simulink model "Almost_there"  (R2022a)
settings: Solver=FixedStepAuto  StartTime=0.0  StopTime=10.0  RelTol=1e-3  EnableMultiTasking=on
undefined symbols (not defined in the file): InputPWM, ticksPerRot, wheelR, WheelSpeed
libraries: arduinolib x19, spsEdgeDetectorLib x2, mobileRoboticsTrainingLib x1
settings Model: ExtModeTrigDuration=2  Creator=heath  LastModifiedBy=noahhavik
settings OptimizationCC: EnhancedBackFolding=on  PassReuseOutputArgsAs=Individual arguments  ZeroExternalMemoryAtStartup=off  ZeroInternalMemoryAtStartup=off  MaxStackSize=64  OptimizeBlockOrder=speed  DifferentSizesBufferReuse=on  OptimizationCustomize=off  EfficientTunableParamExpr=on
settings DebuggingCC: MultiTaskDSMMsg=none  ParameterTunabilityLossMsg=error
settings HardwareCC: ProdBitPerPointer=32  ProdBitPerSizeT=32  ProdBitPerPtrDiffT=32  ProdLargestAtomicInteger=Long  ProdLargestAtomicFloat=Double  ProdWordSize=32  ProdHWDeviceType=ARM Compatible->ARM Cortex  UseEmbeddedCoderFeatures=off  UseSimulinkCoderFeatures=off
settings SFSimCC: MATLABDynamicMemAlloc=off
settings RTWCC: SystemTargetFile=ert.tlc  HardwareBoard=Arduino Nano 33 IoT  TemplateMakefile=ert_default_tmf  Toolchain=Arduino ARM  BuildConfiguration=Faster Runs
settings CodeAppCC: ForceParamTrailComments=on  IgnoreCustomStorageClasses=off  OperatorAnnotations=on  SimulinkDataObjDesc=on  SFDataObjDesc=on  InsertBlockDesc=on
settings ERTTargetCC: SupportContinuousTime=on  SupportNonInlinedSFcns=on  SupportVariableSizeSignals=on  ExtModeTransport=3  ExtModeStaticAlloc=on  ExtModeStaticAllocSize=8192  ExtModeMexFile=ext_xcp  ExtModeIntrfLevel=Level2 - Open

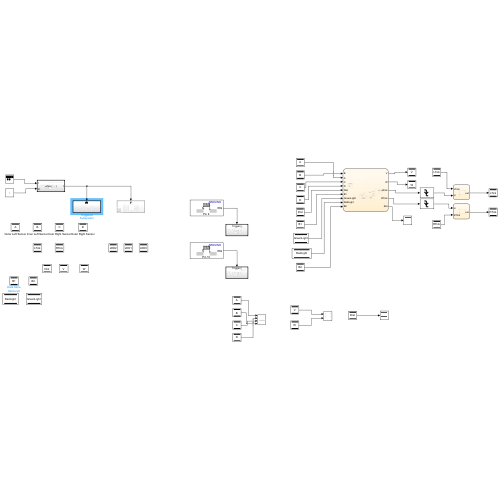
[thumbnail: Simulink's stored preview of the top-level diagram]
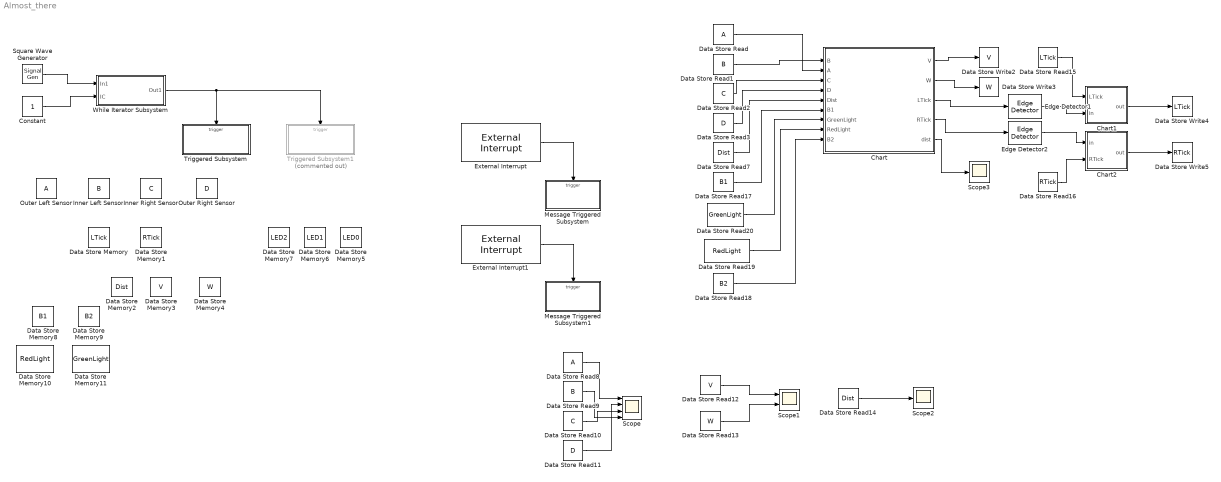
== system Almost_there ==
  Chart : Stateflow chart  TreatAsAtomicUnit=on
  Chart1 : Stateflow chart  TreatAsAtomicUnit=on
  Chart2 : Stateflow chart  TreatAsAtomicUnit=on
  Constant : Constant
  Data Store Memory : DataStoreMemory  DataStoreName=LTick  ShowAdditionalParam=off
  Data Store Memory1 : DataStoreMemory  DataStoreName=RTick  WriteAfterWriteMsg=warning  ShowAdditionalParam=off
  Data Store Memory10 : DataStoreMemory  DataStoreName=RedLight  WriteAfterWriteMsg=warning  ShowAdditionalParam=off
  Data Store Memory11 : DataStoreMemory  DataStoreName=GreenLight  WriteAfterWriteMsg=warning  ShowAdditionalParam=off
  Data Store Memory2 : DataStoreMemory  DataStoreName=Dist  WriteAfterWriteMsg=warning  ShowAdditionalParam=off
  Data Store Memory3 : DataStoreMemory  DataStoreName=V  WriteAfterWriteMsg=warning  ShowAdditionalParam=off
  Data Store Memory4 : DataStoreMemory  DataStoreName=W  WriteAfterWriteMsg=warning  ShowAdditionalParam=off
  Data Store Memory5 : DataStoreMemory  DataStoreName=LED0  WriteAfterWriteMsg=warning  ShowAdditionalParam=off
  Data Store Memory6 : DataStoreMemory  DataStoreName=LED1  WriteAfterWriteMsg=warning  ShowAdditionalParam=off
  Data Store Memory7 : DataStoreMemory  DataStoreName=LED2  WriteAfterWriteMsg=warning  ShowAdditionalParam=off
  Data Store Memory8 : DataStoreMemory  DataStoreName=B1  WriteAfterWriteMsg=warning  ShowAdditionalParam=off
  Data Store Memory9 : DataStoreMemory  DataStoreName=B2  WriteAfterWriteMsg=warning  ShowAdditionalParam=off
  Data Store Read : DataStoreRead  IndexOptions=Index vector (dialog)  Indices=1  OutputSizes=1
  Data Store Read1 : DataStoreRead  DataStoreName=B  IndexOptions=Index vector (dialog)  Indices=1  OutputSizes=1
  Data Store Read10 : DataStoreRead  DataStoreName=C  IndexOptions=Index vector (dialog)  Indices=1  OutputSizes=1
  Data Store Read11 : DataStoreRead  DataStoreName=D  IndexOptions=Index vector (dialog)  Indices=1  OutputSizes=1
  Data Store Read12 : DataStoreRead  DataStoreName=V  IndexOptions=Index vector (dialog)  Indices=1  OutputSizes=1
  Data Store Read13 : DataStoreRead  DataStoreName=W  IndexOptions=Index vector (dialog)  Indices=1  OutputSizes=1
  Data Store Read14 : DataStoreRead  DataStoreName=Dist  IndexOptions=Index vector (dialog)  Indices=1  OutputSizes=1
  Data Store Read15 : DataStoreRead  DataStoreName=LTick  IndexOptions=Index vector (dialog)  Indices=1  OutputSizes=1
  Data Store Read16 : DataStoreRead  DataStoreName=RTick  IndexOptions=Index vector (dialog)  Indices=1  OutputSizes=1
  Data Store Read17 : DataStoreRead  DataStoreName=B1  IndexOptions=Index vector (dialog)  Indices=1  OutputSizes=1
  Data Store Read18 : DataStoreRead  DataStoreName=B2  IndexOptions=Index vector (dialog)  Indices=1  OutputSizes=1
  Data Store Read19 : DataStoreRead  DataStoreName=RedLight  IndexOptions=Index vector (dialog)  Indices=1  OutputSizes=1
  Data Store Read2 : DataStoreRead  DataStoreName=C  IndexOptions=Index vector (dialog)  Indices=1  OutputSizes=1
  Data Store Read20 : DataStoreRead  DataStoreName=GreenLight  IndexOptions=Index vector (dialog)  Indices=1  OutputSizes=1
  Data Store Read3 : DataStoreRead  DataStoreName=D  IndexOptions=Index vector (dialog)  Indices=1  OutputSizes=1
  Data Store Read7 : DataStoreRead  DataStoreName=Dist  IndexOptions=Index vector (dialog)  Indices=1  OutputSizes=1
  Data Store Read8 : DataStoreRead  IndexOptions=Index vector (dialog)  Indices=1  OutputSizes=1
  Data Store Read9 : DataStoreRead  DataStoreName=B  IndexOptions=Index vector (dialog)  Indices=1  OutputSizes=1
  Data Store Write2 : DataStoreWrite  DataStoreName=V  IndexOptions=Index vector (dialog)  Indices=1  OutputSizes=1
  Data Store Write3 : DataStoreWrite  DataStoreName=W  IndexOptions=Index vector (dialog)  Indices=1  OutputSizes=1
  Data Store Write4 : DataStoreWrite  DataStoreName=LTick  IndexOptions=Index vector (dialog)  Indices=1  OutputSizes=1
  Data Store Write5 : DataStoreWrite  DataStoreName=RTick  IndexOptions=Index vector (dialog)  Indices=1  OutputSizes=1
  Edge Detector1 : spsEdgeDetectorLib/Edge Detector  model=Falling  ic=0  Ts=0
      settings: SourceProductBaseCode=PS
  Edge Detector2 : spsEdgeDetectorLib/Edge Detector  model=Falling  ic=0  Ts=0
      settings: SourceProductBaseCode=PS
  External Interrupt : arduinolib/External Interrupt  Pin=9  PullUp=off  Mode=RISING  InterruptSimulationInput=off
      settings: SourceProductBaseCode=ARDUINO
  External Interrupt1 : arduinolib/External Interrupt  Pin=10  PullUp=off  Mode=RISING  InterruptSimulationInput=off
      settings: SourceProductBaseCode=ARDUINO
  Inner Left Sensor : DataStoreMemory  DataStoreName=B  WriteAfterWriteMsg=warning  ShowAdditionalParam=off
  Inner Right Sensor : DataStoreMemory  DataStoreName=C  WriteAfterWriteMsg=warning  ShowAdditionalParam=off
  Message Triggered Subsystem : Subsystem  TreatAsAtomicUnit=on
  Message Triggered Subsystem1 : Subsystem  TreatAsAtomicUnit=on
  Outer Left Sensor : DataStoreMemory  WriteAfterWriteMsg=warning  ShowAdditionalParam=off
  Outer Right Sensor : DataStoreMemory  DataStoreName=D  WriteAfterWriteMsg=warning  ShowAdditionalParam=off
  Scope : Scope  NumInputPorts=4
  Scope1 : Scope  NumInputPorts=2
  Scope2 : Scope
  Scope3 : Scope
  Square Wave Generator : SignalGenerator  WaveForm=square  Frequency=100
  Triggered Subsystem : Subsystem  TreatAsAtomicUnit=on
  Triggered Subsystem1 : Subsystem  Commented=on  TreatAsAtomicUnit=on
  While Iterator Subsystem : Subsystem  TreatAsAtomicUnit=on
  wires:
  Square Wave Generator/1 -> While Iterator Subsystem/1(In1)
  Constant/1 -> While Iterator Subsystem/2(IC)
  External Interrupt/1 -> Message Triggered Subsystem/Trigger
  External Interrupt1/1 -> Message Triggered Subsystem1/Trigger
  While Iterator Subsystem/1(Out1) -> Triggered Subsystem/Trigger, Triggered Subsystem1/Trigger
  Chart/1(V) -> Data Store Write2/1
  Data Store Read7/1 -> Chart/5(Dist)
  Data Store Read3/1 -> Chart/4(D)
  Data Store Read2/1 -> Chart/3(C)
  Data Store Read1/1 -> Chart/1(B)
  Chart/2(W) -> Data Store Write3/1
  Data Store Read/1 -> Chart/2(A)
  Data Store Read8/1 -> Scope/1
  Data Store Read9/1 -> Scope/4
  Data Store Read10/1 -> Scope/3
  Data Store Read11/1 -> Scope/2
  Data Store Read12/1 -> Scope1/1
  Data Store Read13/1 -> Scope1/2
  Data Store Read14/1 -> Scope2/1
  Chart/3(LTick) -> Edge Detector1/1
  Edge Detector1/1 -> Chart1/2(in)
  Chart1/1(out) -> Data Store Write4/1
  Data Store Read15/1 -> Chart1/1(LTick)
  Chart2/1(out) -> Data Store Write5/1
  Edge Detector2/1 -> Chart2/1(in)
  Chart/4(RTick) -> Edge Detector2/1
  Data Store Read16/1 -> Chart2/2(RTick)
  Chart/5(dist) -> Scope3/1
  Data Store Read17/1 -> Chart/6(B1)
  Data Store Read20/1 -> Chart/7(GreenLight)
  Data Store Read19/1 -> Chart/8(RedLight)
  Data Store Read18/1 -> Chart/9(B2)

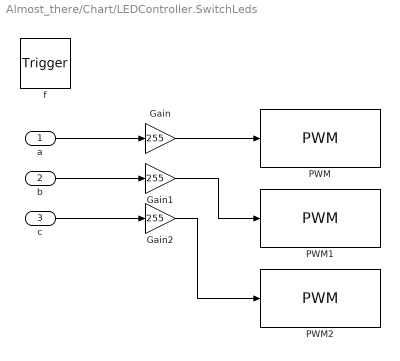
== system Almost_there/Chart/LEDController.SwitchLeds ==
  a : Inport  OutDataTypeStr=double  PortDimensions=1
  b : Inport  Port=2  OutDataTypeStr=double  PortDimensions=1
  c : Inport  Port=3  OutDataTypeStr=double  PortDimensions=1
  f : TriggerPort  TriggerType=function-call  VariantControl=(inherit)
      settings: CopyFcn=Stateflow.SLINSF.SimulinkMan.removeBlockPreDeleteFcn  PreDeleteFcn=Stateflow.SLINSF.SimulinkMan.unsafePredeleteFcn
  Gain : Gain  Gain=255
  Gain1 : Gain  Gain=255
  Gain2 : Gain  Gain=255
  PWM : arduinolib/PWM  pinNumber=16  frequencyType=Default  desiredFrequency=490.2  achievableFrequency=490.2
  PWM1 : arduinolib/PWM  pinNumber=17  frequencyType=Default  desiredFrequency=490.2  achievableFrequency=490.2
  PWM2 : arduinolib/PWM  pinNumber=19  frequencyType=Default  desiredFrequency=490.2  achievableFrequency=490.2
  wires:
  Gain/1 -> PWM/1
  Gain1/1 -> PWM1/1
  Gain2/1 -> PWM2/1
  a/1 -> Gain/1
  b/1 -> Gain1/1
  c/1 -> Gain2/1

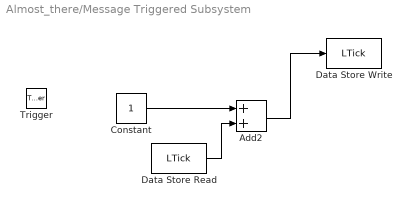
== system Almost_there/Message Triggered Subsystem ==
  Trigger : TriggerPort  TriggerType=function-call  VariantControl=(inherit)  PortDimensions=1
  Add2 : Sum
  Constant : Constant
  Data Store Read : DataStoreRead  DataStoreName=LTick  IndexOptions=Index vector (dialog)  Indices=1  OutputSizes=1
  Data Store Write : DataStoreWrite  DataStoreName=LTick  IndexOptions=Index vector (dialog)  Indices=1  OutputSizes=1
  wires:
  Add2/1 -> Data Store Write/1
  Constant/1 -> Add2/1
  Data Store Read/1 -> Add2/2

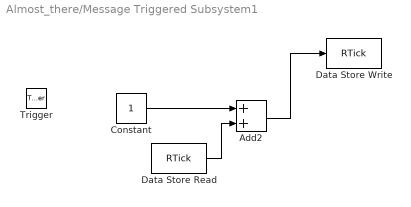
== system Almost_there/Message Triggered Subsystem1 ==
  Trigger : TriggerPort  TriggerType=function-call  VariantControl=(inherit)  PortDimensions=1
  Add2 : Sum
  Constant : Constant
  Data Store Read : DataStoreRead  DataStoreName=RTick  IndexOptions=Index vector (dialog)  Indices=1  OutputSizes=1
  Data Store Write : DataStoreWrite  DataStoreName=RTick  IndexOptions=Index vector (dialog)  Indices=1  OutputSizes=1
  wires:
  Add2/1 -> Data Store Write/1
  Constant/1 -> Add2/1
  Data Store Read/1 -> Add2/2

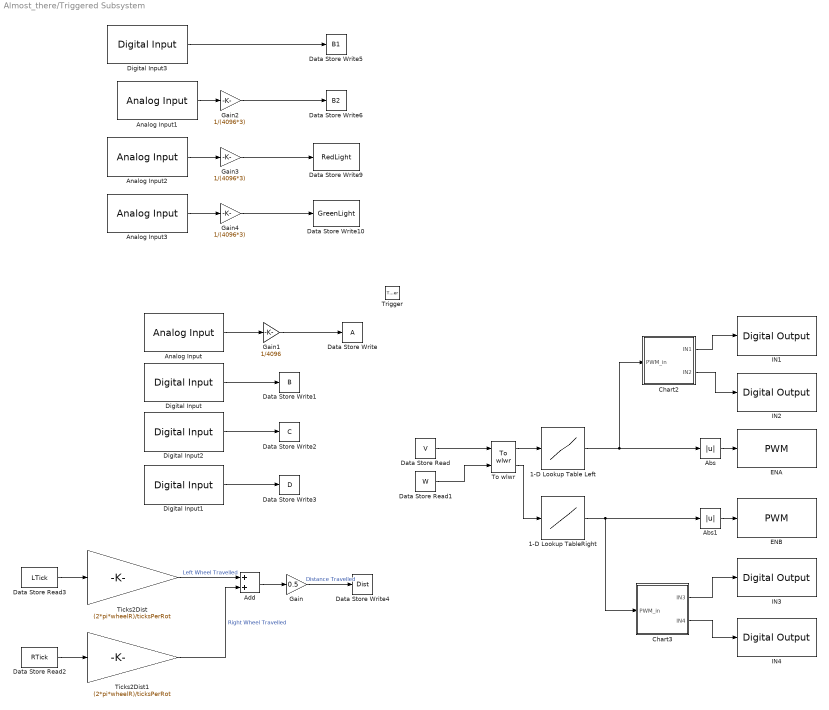
== system Almost_there/Triggered Subsystem ==
  Trigger : TriggerPort  TriggerType=either  VariantControl=(inherit)
  1-D Lookup Table Left : Lookup_n-D  NumberOfTableDimensions=1  BreakpointsForDimension1=WheelSpeed  Table=InputPWM  InternalRulePriority=Speed  RndMeth=Simplest
  1-D Lookup TableRight : Lookup_n-D  NumberOfTableDimensions=1  BreakpointsForDimension1=WheelSpeed  Table=InputPWM  InternalRulePriority=Speed  RndMeth=Simplest
  Abs : Abs  SaturateOnIntegerOverflow=off
  Abs1 : Abs  SaturateOnIntegerOverflow=off
  Add : Sum
  Analog Input : arduinolib/Analog Input  pinNumber=0  ReadResultsOnly=off  ConversionTriggerSource=Software  ExternalTriggerType=uint32( 0 )  OutputDataType=uint16  EnableConversionCompleteNotify=off  EnableOuputStatus=off  SampleTime=-1  blockPlatform=arduino
  Analog Input1 : arduinolib/Analog Input  pinNumber=1  ReadResultsOnly=off  ConversionTriggerSource=Software  ExternalTriggerType=uint32( 0 )  OutputDataType=uint16  EnableConversionCompleteNotify=off  EnableOuputStatus=off  SampleTime=-1  blockPlatform=arduino
  Analog Input2 : arduinolib/Analog Input  pinNumber=6  ReadResultsOnly=off  ConversionTriggerSource=Software  ExternalTriggerType=uint32( 0 )  OutputDataType=uint16  EnableConversionCompleteNotify=off  EnableOuputStatus=off  SampleTime=-1  blockPlatform=arduino
  Analog Input3 : arduinolib/Analog Input  pinNumber=7  ReadResultsOnly=off  ConversionTriggerSource=Software  ExternalTriggerType=uint32( 0 )  OutputDataType=uint16  EnableConversionCompleteNotify=off  EnableOuputStatus=off  SampleTime=-1  blockPlatform=arduino
  Chart2 : Stateflow chart  TreatAsAtomicUnit=on
  Chart3 : Stateflow chart  TreatAsAtomicUnit=on
  Data Store Read : DataStoreRead  DataStoreName=V  IndexOptions=Index vector (dialog)  Indices=1  OutputSizes=1
  Data Store Read1 : DataStoreRead  DataStoreName=W  IndexOptions=Index vector (dialog)  Indices=1  OutputSizes=1
  Data Store Read2 : DataStoreRead  DataStoreName=RTick  IndexOptions=Index vector (dialog)  Indices=1  OutputSizes=1
  Data Store Read3 : DataStoreRead  DataStoreName=LTick  IndexOptions=Index vector (dialog)  Indices=1  OutputSizes=1
  Data Store Write : DataStoreWrite  IndexOptions=Index vector (dialog)  Indices=1  OutputSizes=1
  Data Store Write1 : DataStoreWrite  DataStoreName=B  IndexOptions=Index vector (dialog)  Indices=1  OutputSizes=1
  Data Store Write10 : DataStoreWrite  DataStoreName=GreenLight  IndexOptions=Index vector (dialog)  Indices=1  OutputSizes=1
  Data Store Write2 : DataStoreWrite  DataStoreName=C  IndexOptions=Index vector (dialog)  Indices=1  OutputSizes=1
  Data Store Write3 : DataStoreWrite  DataStoreName=D  IndexOptions=Index vector (dialog)  Indices=1  OutputSizes=1
  Data Store Write4 : DataStoreWrite  DataStoreName=Dist  IndexOptions=Index vector (dialog)  Indices=1  OutputSizes=1
  Data Store Write5 : DataStoreWrite  DataStoreName=B1  IndexOptions=Index vector (dialog)  Indices=1  OutputSizes=1
  Data Store Write6 : DataStoreWrite  DataStoreName=B2  IndexOptions=Index vector (dialog)  Indices=1  OutputSizes=1
  Data Store Write9 : DataStoreWrite  DataStoreName=RedLight  IndexOptions=Index vector (dialog)  Indices=1  OutputSizes=1
  Digital Input : arduinolib/Digital Input  pinNumber=12  mode=Default  Direction=input  SampleTime=-1  blockPlatform=arduino
  Digital Input1 : arduinolib/Digital Input  pinNumber=8  mode=Default  Direction=input  SampleTime=-1  blockPlatform=arduino
  Digital Input2 : arduinolib/Digital Input  pinNumber=11  mode=Default  Direction=input  SampleTime=-1  blockPlatform=arduino
  Digital Input3 : arduinolib/Digital Input  pinNumber=13  mode=Default  Direction=input  SampleTime=-1  blockPlatform=arduino
  ENA : arduinolib/PWM  pinNumber=3  frequencyType=Default  desiredFrequency=490.2  achievableFrequency=490.2
  ENB : arduinolib/PWM  pinNumber=2  frequencyType=Default  desiredFrequency=490.2  achievableFrequency=490.2
  Gain : Gain  Gain=0.5
  Gain1 : Gain  Gain=1/4096
  Gain2 : Gain  Gain=1/(4096*3)
  Gain3 : Gain  Gain=1/(4096*3)
  Gain4 : Gain  Gain=1/(4096*3)
  IN1 : arduinolib/Digital Output  pinNumber=4  Direction=output  blockPlatform=arduino
  IN2 : arduinolib/Digital Output  pinNumber=5  Direction=output  blockPlatform=arduino
  IN3 : arduinolib/Digital Output  pinNumber=6  Direction=output  blockPlatform=arduino
  IN4 : arduinolib/Digital Output  pinNumber=7  Direction=output  blockPlatform=arduino
  Ticks2Dist : Gain  Gain=(2*pi*wheelR)/ticksPerRot
  Ticks2Dist1 : Gain  Gain=(2*pi*wheelR)/ticksPerRot
  To wlwr : mobileRoboticsTrainingLib/To wlwr  axleLength=axleLength  wheelR=wheelR
  wires:
  Chart3/2(IN4) -> IN4/1
  Chart2/2(IN2) -> IN2/1
  Chart2/1(IN1) -> IN1/1
  Abs1/1 -> ENB/1
  Abs/1 -> ENA/1
  1-D Lookup TableRight/1 -> Chart3/1(PWM_in), Abs1/1
  Chart3/1(IN3) -> IN3/1
  To wlwr/2 -> 1-D Lookup TableRight/1
  To wlwr/1 -> 1-D Lookup Table Left/1
  1-D Lookup Table Left/1 -> Chart2/1(PWM_in), Abs/1
  Data Store Read/1 -> To wlwr/1
  Data Store Read1/1 -> To wlwr/2
  Analog Input/1 -> Gain1/1
  Digital Input/1 -> Data Store Write1/1
  Digital Input2/1 -> Data Store Write2/1
  Digital Input1/1 -> Data Store Write3/1
  Data Store Read3/1 -> Ticks2Dist/1
  Ticks2Dist/1 -> Add/1  "Left Wheel Travelled"
  Data Store Read2/1 -> Ticks2Dist1/1
  Add/1 -> Gain/1
  Ticks2Dist1/1 -> Add/2  "Right Wheel Travelled"
  Gain/1 -> Data Store Write4/1  "Distance Travelled"
  Gain1/1 -> Data Store Write/1
  Digital Input3/1 -> Data Store Write5/1
  Gain2/1 -> Data Store Write6/1
  Gain4/1 -> Data Store Write10/1
  Gain3/1 -> Data Store Write9/1
  Analog Input1/1 -> Gain2/1
  Analog Input2/1 -> Gain3/1
  Analog Input3/1 -> Gain4/1

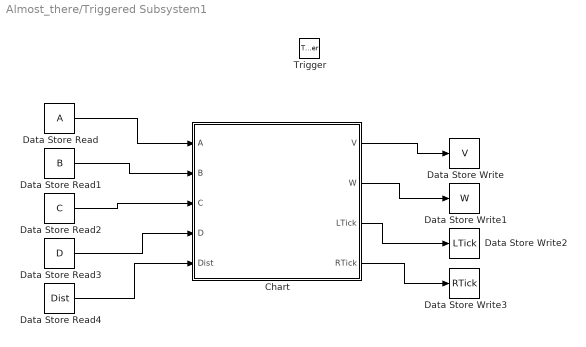
== system Almost_there/Triggered Subsystem1 ==
  Trigger : TriggerPort  VariantControl=(inherit)
  Chart : Stateflow chart  TreatAsAtomicUnit=on
      settings: PortSchema="{\"entries\":[{\"content\":{\"sides\":[{\"content\":{\"connectorIds\":[\"In2\",\"In1\",\"In3\",\"In4\",\"In5\"]},\"type\":\"ConnectorPlacement.EquallySpacedRectSide\",\"uuid\":\"bce85c3e-dc0f-4a3e-9298-fc19bb09231c\"},{\"content\":{\"connectorIds\":[\"Out1\",\"Out2\",\"Out3\",\"Out4\"],\"side\":\"RIGHT\"},\"type\":\"ConnectorPlacement.EquallySpacedRectSide\",\"uuid\":\"1feae271-0488-4834-a59c-2ee78774caf2\"},{\"content\":{\"connectorIds\":[],\"side\":\"TOP\"},\"type\":\"ConnectorPlacement.EquallySpacedRectSide\",\"uuid\":\"1d04e7bd-f523-4552-a513-f16d21fd726a\"}]},\"type\":\"ConnectorPlacement.EquallySpacedConnector\",\"uuid\":\"4fe39406-b24c-4b02-90d6-d6f48c1deb78\"}],\"packageUris\":[\"http://schema.mathworks.com/mf0/Connector/R2020b\"],\"version\":\"1.0\"}"
  Data Store Read : DataStoreRead  IndexOptions=Index vector (dialog)  Indices=1  OutputSizes=1
  Data Store Read1 : DataStoreRead  DataStoreName=B  IndexOptions=Index vector (dialog)  Indices=1  OutputSizes=1
  Data Store Read2 : DataStoreRead  DataStoreName=C  IndexOptions=Index vector (dialog)  Indices=1  OutputSizes=1
  Data Store Read3 : DataStoreRead  DataStoreName=D  IndexOptions=Index vector (dialog)  Indices=1  OutputSizes=1
  Data Store Read4 : DataStoreRead  DataStoreName=Dist  IndexOptions=Index vector (dialog)  Indices=1  OutputSizes=1
  Data Store Write : DataStoreWrite  DataStoreName=V  IndexOptions=Index vector (dialog)  Indices=1  OutputSizes=1
  Data Store Write1 : DataStoreWrite  DataStoreName=W  IndexOptions=Index vector (dialog)  Indices=1  OutputSizes=1
  Data Store Write2 : DataStoreWrite  DataStoreName=LTick  IndexOptions=Index vector (dialog)  Indices=1  OutputSizes=1
  Data Store Write3 : DataStoreWrite  DataStoreName=RTick  IndexOptions=Index vector (dialog)  Indices=1  OutputSizes=1
  wires:
  Data Store Read/1 -> Chart/2(A)
  Data Store Read1/1 -> Chart/1(B)
  Data Store Read2/1 -> Chart/3(C)
  Data Store Read3/1 -> Chart/4(D)
  Data Store Read4/1 -> Chart/5(Dist)
  Chart/1(V) -> Data Store Write/1
  Chart/2(W) -> Data Store Write1/1
  Chart/3(LTick) -> Data Store Write2/1
  Chart/4(RTick) -> Data Store Write3/1

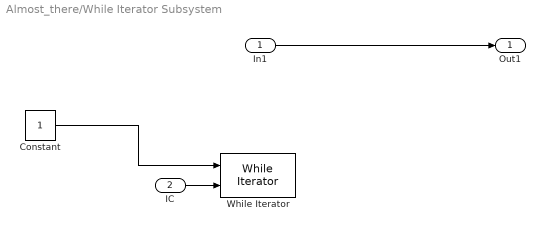
== system Almost_there/While Iterator Subsystem ==
  In1 : Inport
  IC : Inport  Port=2
  Constant : Constant
  While Iterator : WhileIterator
  Out1 : Outport
  wires:
  IC/1 -> While Iterator/2
  In1/1 -> Out1/1
  Constant/1 -> While Iterator/1

== stateflow chart Almost_there/Chart ==
  settings: updateMethod=CONTINUOUS
  state Initial [commented out]
    entry:
    W = 0;
    V = 0;
    LEDController.SetLEDState(LEDStates.IDLE);
  state LEDController [group]
    state SwitchLeds(a,b,c) [function]
  state WaitForLight [commented out]
    entry:
    LEDController.SetLEDState(LEDStates.WAITINGFORLIGHT);
  state WaitForGreen [commented out]
    entry:
    LEDController.SetLEDState(LEDStates.SENSINGRED);
  state WaitForStart [commented out]
    entry:
    LEDController.SetLEDState(LEDStates.SENSINGGREEN);
  state Stop
    entry:
    done=0;
    V = 0;
    W = 0;
  state Find_Line
    entry:
    done = 0;
    state Found
      entry:
      done=1;
    state Finding_line
      entry:
      V=0.13;
    (default) -> Finding_line
    Finding_line -> Found : [B<0.5||C<0.5]
  state Turn_right_90
    entry:
    done = 0;
    cblack = 0;
    target = (pi*0.136/4);
    LTick=0;RTick=0;
    state cblack_increment
      entry:
      cblack = cblack + 1;
    state Turn
      entry:
      V=0;
      W = -1.5;
      during:
      dist = Dist;
    state Stop1
      entry:
      done=1;
      during:
      dist = Dist;
    Turn_right_90.Turn -> Turn_right_90.cblack_increment [order 2] : [C<0.5]
    Turn_right_90.cblack_increment -> Turn_right_90.Turn : [C>0.5]
    (default) -> Turn_right_90.Turn
    Turn_right_90.Turn -> Turn_right_90.Stop1 [order 1] : [cblack==2]
  state Drive_1cm_3
    entry:
    done = 0;
    target = 0.02;
    LTick=0;RTick=0;
    exit:
    LTick = 1;RTick=1;
    state Stop
      entry:
      done=1;
      during:
      dist = Dist;
    state forward_1cm
      entry:
      V = 0.13;
      W = 0;
      during:
      dist = Dist;
    Drive_1cm_3.forward_1cm -> Drive_1cm_3.Stop : [Dist>target]
    (default) -> Drive_1cm_3.forward_1cm
  state Drive_1cm_4
    entry:
    done = 0;
    target = 0.013;
    LTick=0;RTick=0;
    exit:
    LTick=1;RTick=1;
    state Stop1
      entry:
      done=1;
      during:
      dist = Dist;
    state forward_1cm
      entry:
      V = 0.13;
      W = 0;
      during:
      dist = Dist;
    (default) -> Drive_1cm_4.forward_1cm
    Drive_1cm_4.forward_1cm -> Drive_1cm_4.Stop1 : [Dist>target]
  state Follow_Line
    entry:
    V=0.13;
    W=0;
    %LEDController.SetLEDState(LEDStates.ENDOFMAZE);
    LTick=1;RTick=1;done=0;
  state Drive_1cm_2
    entry:
    done = 0;
    target = 0.02;
    LTick=0;RTick=0;
    exit:
    LTick=1;RTick=1;
    state Stop
      entry:
      done=1;
      during:
      dist = Dist;
    state forward_1cm
      entry:
      V = 0.13;
      W = 0;
      during:
      dist = Dist;
    (default) -> Drive_1cm_2.forward_1cm
    Drive_1cm_2.forward_1cm -> Drive_1cm_2.Stop : [Dist>target]
  state Turn_right_91
    entry:
    done = 0;
    cblack = 0;
    target = (pi*0.136/4);
    LTick=0;RTick=0;
    state cblack_increment
      entry:
      cblack = cblack + 1;
    state Turn
      entry:
      V=0;
      W = -1.5;
      during:
      dist = Dist;
    state Stop1
      entry:
      done=1;
      during:
      dist = Dist;
    Turn_right_91.Turn -> Turn_right_91.cblack_increment [order 2] : [C<0.5]
    Turn_right_91.cblack_increment -> Turn_right_91.Turn : [C>0.5]
    (default) -> Turn_right_91.Turn
    Turn_right_91.Turn -> Turn_right_91.Stop1 [order 1] : [cblack==1]
  state Drive_1cm_5
    entry:
    done = 0;
    target = 0.02;
    LTick=0;RTick=0;
    exit:
    LTick = 1;RTick = 1;
    state Stop
      entry:
      done=1;
      during:
      dist = Dist;
    state forward_1cm
      entry:
      V = 0.13;
      W = 0;
      during:
      dist = Dist;
    (default) -> Drive_1cm_5.forward_1cm
    Drive_1cm_5.forward_1cm -> Drive_1cm_5.Stop : [Dist>target]
  state Drive_1cm
    entry:
    done = 0;
    target = 0.02;
    LTick=0;RTick=0;
    exit:
    LTick = 1;RTick = 1;
    state Stop
      entry:
      done=1;
      during:
      dist = Dist;
    state forward_1cm
      entry:
      V = 0.13;
      W = 0;
      during:
      dist = Dist;
    (default) -> Drive_1cm.forward_1cm
    Drive_1cm.forward_1cm -> Drive_1cm.Stop : [Dist>target]
  state Turn_180
    entry:
    done = 0;
    target = (pi*0.136/2);
    LTick=0;RTick=0;
    state Turn
      entry:
      V=0;
      W = 1.5;
      during:
      dist = Dist;
    state Stop
      entry:
      done=1;
      during:
      dist = Dist;
    (default) -> Turn_180.Turn
    Turn_180.Turn -> Turn_180.Stop : [B<0.5]
  state Turn_right
    entry:
    done=0;
    V = 0.13;
    W = 1.5;
    done=1;
  state Turn_left
    entry:
    done=0;
    V = 0.13;
    W = -1.5;
    done=1;
  state Turn_Left_90
    entry:
    done = 0;
    target = (pi*0.136/4);
    LTick=0;RTick=0;
    state Stop1
      entry:
      done=1;
      during:
      dist = Dist;
    state Turn
      entry:
      V=0;
      W = 1.5;
      during:
      dist = Dist;
    (default) -> Turn_Left_90.Turn
    Turn_Left_90.Turn -> Turn_Left_90.Stop1 : [B<0.5]
  Initial -> WaitForLight [commented out] : [B1 > 0]
  WaitForLight -> WaitForGreen [commented out] : [RedLight > 0.5]
  WaitForGreen -> WaitForLight [commented out] : [RedLight < 0.5]
  WaitForGreen -> WaitForStart [commented out] : [GreenLight > 0.5]
  WaitForStart -> WaitForGreen [commented out] : [GreenLight < 0.5]
  WaitForStart -> Follow_Line [commented out] : [B2 > 0.5]
  Drive_1cm_3 -> Stop [order 1] : [A<0.5&&B<0.5&&C<0.5&&D<0.5&&done==1]
  Drive_1cm_3 -> Find_Line [order 3] : [A>0.5&&B>0.5&&C>0.5&&D>0.5&&done==1]
  Find_Line -> Follow_Line : [done==1]
  Drive_1cm_3 -> Turn_right_90 [order 2] : [A>0.5&&B<0.5&&C<0.5&&D>0.5&&done==1]
  Drive_1cm_4 -> Drive_1cm_2 [order 1] : [A>0.5&&D<0.5&&done==1]
  Follow_Line -> Drive_1cm_4 [order 4] : [A<0.5||D<0.5]
  Turn_right_90 -> Follow_Line : [done==1]
  (default) -> Follow_Line
  Drive_1cm_4 -> Drive_1cm_3 [order 3] : [A<0.5&&D<0.5&&done==1]
  Drive_1cm_4 -> Drive_1cm [order 2] : [A<0.5&&D>0.5&&done==1]
  Turn_Left_90 -> Follow_Line : [done==1]
  Turn_left -> Follow_Line : [done==1]
  Turn_right -> Follow_Line : [done==1]
  Follow_Line -> Turn_left [order 2] : [B<0.5&&C>0.5]
  Drive_1cm_2 -> Turn_right_91 : [done==1]
  Follow_Line -> Drive_1cm_5 [order 1] : [A>0.5&&B>0.5&&C>0.5&&D>0.5]
  Turn_180 -> Follow_Line : [done==1]
  Follow_Line -> Turn_right [order 3] : [B>0.5&&C<0.5]
  Turn_right_91 -> Follow_Line : [done==1]
  Drive_1cm -> Follow_Line [order 2] : [B<0.5&&C<0.5&&done==1]
  Drive_1cm -> Turn_Left_90 [order 1] : [B>0.5&&C>0.5&&done==1]
  Drive_1cm_5 -> Turn_180 : [done==1]
  data: state function_input Enum: LEDStates; a function_input double size=1; b function_input double size=1; c function_input double size=1; B input; A input; C input; D input; Dist input; V output; W output; done local; target local; LTick output; RTick output; dist output; B1 input; GreenLight input; RedLight input; B2 input; cblack local
  function SetLEDState(state):
    | function SetLEDState(state)
    |     one = bitshift(state, -2) & 1;
    |     two = bitshift(state, -1) & 1;
    |     % Useless bitshift to remove errors
    |     three = bitshift(state, 0) & 1;
    |     SwitchLeds(one, two,three);
    | 
    | end

== stateflow chart Almost_there/Triggered Subsystem/Chart2 ==
  state Forward
    entry:
    IN1 = 1;
    IN2 = 0;
  state Back
    entry:
    IN1 = 0;
    IN2 = 1;
  (default) -> Forward
  Forward -> Back : [PWM_in<0]
  Back -> Forward : [PWM_in>=0]
  data: PWM_in input; IN1 output; IN2 output

== stateflow chart Almost_there/Triggered Subsystem1/Chart ==
  state Follow_Line
  state Drive_1cm_2
    entry:
    done = 0;
  state Drive_1cm
    entry:
    done = 0;
  state Stop
  state Turn_180
    entry:
    done = 0;
  state Drive
    entry:
    done = 0;
  state Turn_right
    entry:
    done = 0;
  state Turn_left
    entry:
    done = 0;
  state Turn_Left_90
    entry:
    done = 0;
  state Turn_right_90
    entry:
    done = 0;
  state Find_Line
    entry:
    done = 0;
  Follow_Line -> Drive_1cm_2 [order 2] : [A<0.5&&D<0.5]
  (default) -> Follow_Line
  Find_Line -> Follow_Line : [done==1]
  Turn_right_90 -> Follow_Line : [done==1]
  Follow_Line -> Turn_right_90 [order 3] : [A>0.5&&D<0.5]
  Turn_Left_90 -> Follow_Line : [done==1]
  Turn_left -> Follow_Line : [done==1]
  Turn_right -> Follow_Line : [done==1]
  Follow_Line -> Turn_left [order 5] : [B<0.5&&C>0.5]
  Drive_1cm_2 -> Stop [order 3] : [A<0.5&&B<0.5&&C<0.5&&D<0.5&&done==1]
  Drive_1cm_2 -> Find_Line [order 2] : [A>0.5&&B>0.5&&C>0.5&&D>0.5&&done==1]
  Follow_Line -> Drive_1cm [order 4] : [A<0.5&&D>0.5]
  Drive_1cm_2 -> Turn_right_90 [order 1] : [A>0.5&&B<0.5&&C<0.5&&D>0.5&&done==1]
  Turn_180 -> Follow_Line : [done==1]
  Follow_Line -> Turn_180 [order 1] : [A>0.5&&B>0.5&&C>0.5&&D>0.5]
  Follow_Line -> Drive [order 7] : [B<0.5&&C<0.5]
  Drive -> Follow_Line : [done==1]
  Follow_Line -> Turn_right [order 6] : [B>0.5&&C<0.5]
  Drive_1cm -> Drive [order 2] : [B<0.5&&C<0.5&&done==1]
  Drive_1cm -> Turn_Left_90 [order 1] : [B>0.5&&C>0.5&&done==1]
  data: B input; A input; C input; D input; Dist input; V output; W output; LTick output; RTick output

== stateflow chart Almost_there/Triggered Subsystem/Chart3 ==
  state Forward
    entry:
    IN4 = 0;
    IN3 = 1;
  state Back
    entry:
    IN4 = 1;
    IN3 = 0;
  (default) -> Forward
  Forward -> Back : [PWM_in<0]
  Back -> Forward : [PWM_in>=0]
  data: PWM_in input; IN3 output; IN4 output

== stateflow chart Almost_there/Chart1 ==
  (default) -> (junction 8)
  (junction 8) -> (junction 9) [order 1] : [in]
  (junction 8) -> (junction 10) [order 2] : {out = LTick}
  (junction 9) -> (junction 11) : {out = 0;}
  (junction 11) -> (junction 10)
  (junction 10) -> (junction 12)
  data: LTick input; in input; out output

== stateflow chart Almost_there/Chart2 ==
  (default) -> (junction 8)
  (junction 8) -> (junction 9) [order 1] : [in]
  (junction 8) -> (junction 10) [order 2] : {out = RTick}
  (junction 9) -> (junction 11) : {out = 0;}
  (junction 11) -> (junction 10)
  (junction 10) -> (junction 12)
  data: in input; out output; RTick input
